simulink model "inv_mod"  (R2022b)
settings: Solver=ode3  StartTime=0.0  StopTime=2  FixedStep=1.6666666851961055e-7  RelTol=1e-3
libraries: spsIGBTDiodeLib x4, spsSeriesRLCBranchLib x3, simulink x2, spsVoltageMeasurementLib x2, spsGroundLib x1, spsCurrentMeasurementLib x1, spsDCVoltageSourceLib x1, spspowerguiLib x1
settings Model: Creator=76475  LastModifiedBy=76475
settings DataIOCC: ReturnWorkspaceOutputs=off

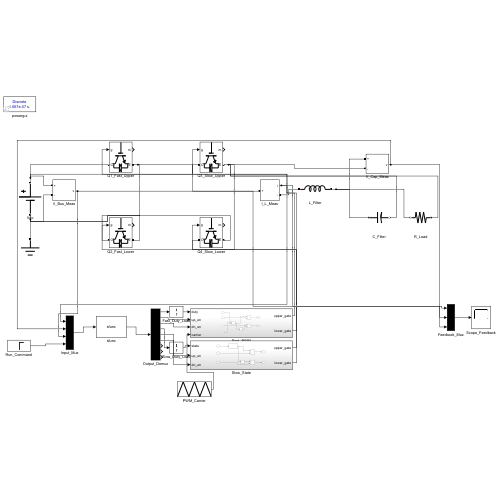
[thumbnail: Simulink's stored preview of the top-level diagram]
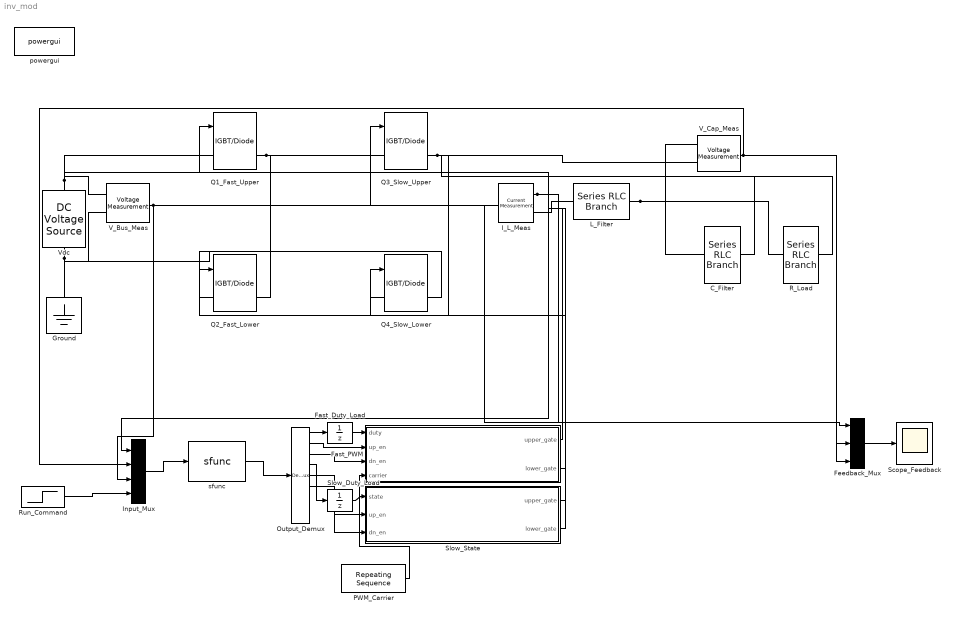
== system inv_mod ==
  C_Filter : spsSeriesRLCBranchLib/Series RLC Branch  LConnTagsString=__new0  RConnTagsString=__new0  BranchType=C  Resistance=1  Inductance=1e-3  SetiL0=off  InitialCurrent=0  Capacitance=12e-6  Setx0=off  InitialVoltage=0  Measurements=None
  Fast_Duty_Load : UnitDelay  SampleTime=3.3333333703922108e-5  HasFrameUpgradeWarning=on
  Fast_PWM : Subsystem
  Feedback_Mux : Mux  Inputs=3
  Ground : spsGroundLib/Ground  LConnTagsString=a
  I_L_Meas : spsCurrentMeasurementLib/Current Measurement  PhasorSimulation=off  OutputType=Complex  PSBequivalent=0
  Input_Mux : Mux
  L_Filter : spsSeriesRLCBranchLib/Series RLC Branch  LConnTagsString=__new0  RConnTagsString=__new0  BranchType=L  Resistance=0.05  Inductance=440e-6  SetiL0=off  InitialCurrent=0  Capacitance=1e-6  Setx0=off  InitialVoltage=0  Measurements=None
  Output_Demux : Demux  Outputs=[1 1 1 1 1 1 1 1 22]
  PWM_Carrier : simulink/Sources/Repeating Sequence  rep_seq_t=[0 1.6666666851961054e-5 3.3333333703922108e-5]  rep_seq_y=[0 1 0]
  Q1_Fast_Upper : spsIGBTDiodeLib/IGBT//Diode  Ron=1e-3  Rs=1e5  Cs=inf  Measurements=on
  Q2_Fast_Lower : spsIGBTDiodeLib/IGBT//Diode  Ron=1e-3  Rs=1e5  Cs=inf  Measurements=on
  Q3_Slow_Upper : spsIGBTDiodeLib/IGBT//Diode  Ron=1e-3  Rs=1e5  Cs=inf  Measurements=on
  Q4_Slow_Lower : spsIGBTDiodeLib/IGBT//Diode  Ron=1e-3  Rs=1e5  Cs=inf  Measurements=on
  R_Load : spsSeriesRLCBranchLib/Series RLC Branch  LConnTagsString=__new0  RConnTagsString=__new0  BranchType=R  Resistance=220  Inductance=1e-3  SetiL0=off  InitialCurrent=0  Capacitance=1e-6  Setx0=off  InitialVoltage=0  Measurements=None
  Run_Command : Step  Time=0.02  SampleTime=0
  Scope_Feedback : Scope
  Slow_Duty_Load : UnitDelay  SampleTime=3.3333333703922108e-5  HasFrameUpgradeWarning=on
  Slow_State : Subsystem
  V_Bus_Meas : spsVoltageMeasurementLib/Voltage Measurement  PhasorSimulation=off  OutputType=Complex  PSBequivalent=0
  V_Cap_Meas : spsVoltageMeasurementLib/Voltage Measurement  PhasorSimulation=off  OutputType=Complex  PSBequivalent=0
  Vdc : spsDCVoltageSourceLib/DC Voltage Source  Amplitude=400  Measurements=None
  powergui : spspowerguiLib/powergui  Priority=1  SimulationMode=Discrete  SampleTime=1.6666666851961055e-7  frequency=60  Iterations=50  frequencyindice=0  Pbase=100e6  ErrMax=1e-4  UnitsV=kV  UnitsW=MW  buscounter=0  FunctionMessages=off  echomessages=off  EnableUseOfTLC=off  CurrentSourceSwitches=off  DisableSnubberDevices=off  DisableRonSwitches=off  DisableVfSwitches=off  DisplayEquations=off  AutomaticDiscreteSolvers=off  SolverType=Tustin/Backward Euler (TBE)  Interpol=off  ExternalGateDelay=off  methode=off  Ts=100  x0status=blocks  SPID=on  SwTol=0  HookPort=off  NonlinearTolerance=1e-4  nMaxIteration=100  ContinueOnMaxIteration=off  RestoreLinks=warning  ResistiveCurrentMeasurement=off  Frange=[0:2:500]  Ylog=off  Xlog=on  ShowGrid=off  save=off  variable=ZData  structure=0  ZoomFFT=off  StartTime=0.0  cycles=1  DisplayStyle=1  fundamental=60  FreqAxis=off  MaxFrequency=1000  frequencyindicesteady=1  RmsSteady=1  display=off
  sfunc : S-Function  FunctionName=sfunc  SFunctionDeploymentMode=off  EnableBusSupport=off
  wires:
  I_L_Meas/1 -> Input_Mux/1, Feedback_Mux/1
  V_Cap_Meas/1 -> Input_Mux/2, Feedback_Mux/2
  V_Bus_Meas/1 -> Input_Mux/3, Feedback_Mux/3
  Run_Command/1 -> Input_Mux/4
  Input_Mux/1 -> sfunc/1
  sfunc/1 -> Output_Demux/1
  Output_Demux/1 -> Fast_Duty_Load/1
  Fast_Duty_Load/1 -> Fast_PWM/1(duty)
  Output_Demux/2 -> Fast_PWM/2(up_en)
  Output_Demux/3 -> Fast_PWM/3(dn_en)
  PWM_Carrier/1 -> Fast_PWM/4(carrier)
  Fast_PWM/1(upper_gate) -> Q1_Fast_Upper/1
  Fast_PWM/2(lower_gate) -> Q2_Fast_Lower/1
  Output_Demux/4 -> Slow_Duty_Load/1
  Slow_Duty_Load/1 -> Slow_State/1(state)
  Output_Demux/5 -> Slow_State/2(up_en)
  Output_Demux/6 -> Slow_State/3(dn_en)
  Slow_State/1(upper_gate) -> Q3_Slow_Upper/1
  Slow_State/2(lower_gate) -> Q4_Slow_Lower/1
  Feedback_Mux/1 -> Scope_Feedback/1
  connections:
  Q1_Fast_Upper/LConn1 -- Vdc/RConn1 -- Q3_Slow_Upper/LConn1 -- V_Bus_Meas/LConn1
  Q2_Fast_Lower/RConn1 -- Vdc/LConn1 -- Q4_Slow_Lower/RConn1 -- Ground/LConn1 -- V_Bus_Meas/LConn2
  Q2_Fast_Lower/LConn1 -- Q1_Fast_Upper/RConn1 -- I_L_Meas/LConn1
  Q4_Slow_Lower/LConn1 -- Q3_Slow_Upper/RConn1 -- C_Filter/RConn1 -- R_Load/RConn1 -- V_Cap_Meas/LConn2
  I_L_Meas/RConn1 -- L_Filter/LConn1
  C_Filter/LConn1 -- L_Filter/RConn1 -- R_Load/LConn1 -- V_Cap_Meas/LConn1

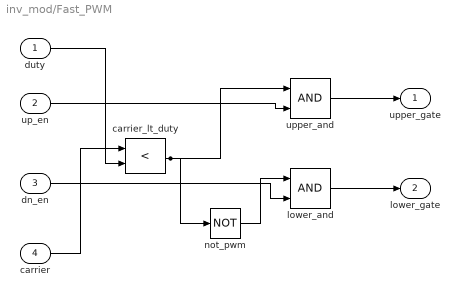
== system inv_mod/Fast_PWM ==
  duty : Inport
  up_en : Inport  Port=2
  dn_en : Inport  Port=3
  carrier : Inport  Port=4
  carrier_lt_duty : RelationalOperator  Operator=<  OutDataTypeStr=boolean  RndMeth=Simplest  InputSameDT=off
  lower_and : Logic  AllPortsSameDT=off  OutDataTypeStr=boolean
  not_pwm : Logic  Operator=NOT  AllPortsSameDT=off  OutDataTypeStr=boolean
  upper_and : Logic  AllPortsSameDT=off  OutDataTypeStr=boolean
  upper_gate : Outport
  lower_gate : Outport  Port=2
  wires:
  carrier/1 -> carrier_lt_duty/1
  duty/1 -> carrier_lt_duty/2
  carrier_lt_duty/1 -> upper_and/1, not_pwm/1
  up_en/1 -> upper_and/2
  not_pwm/1 -> lower_and/1
  dn_en/1 -> lower_and/2
  upper_and/1 -> upper_gate/1
  lower_and/1 -> lower_gate/1

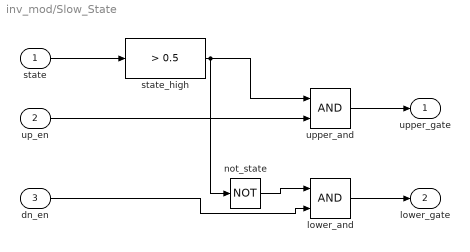
== system inv_mod/Slow_State ==
  state : Inport
  up_en : Inport  Port=2
  dn_en : Inport  Port=3
  lower_and : Logic  AllPortsSameDT=off  OutDataTypeStr=boolean
  not_state : Logic  Operator=NOT  AllPortsSameDT=off  OutDataTypeStr=boolean
  state_high : simulink/Logic and Bit Operations/Compare To Constant  relop=>  const=0.5  OutDataTypeStr=boolean
  upper_and : Logic  AllPortsSameDT=off  OutDataTypeStr=boolean
  upper_gate : Outport
  lower_gate : Outport  Port=2
  wires:
  state/1 -> state_high/1
  state_high/1 -> upper_and/1, not_state/1
  up_en/1 -> upper_and/2
  not_state/1 -> lower_and/1
  dn_en/1 -> lower_and/2
  upper_and/1 -> upper_gate/1
  lower_and/1 -> lower_gate/1
